simulink model "Virtual"  (Simulink 8.6)
settings: Solver=ode45  StartTime=0.0  StopTime=50.0  RelTol=1e-3
settings Model: Creator=Nasir  LastModifiedBy=Nasir
settings DebuggingCC: FcnCallInpInsideContextMsg=UseLocalSettings  StrictBusMsg=Warning
settings GRTTargetCC: GeneratePreprocessorConditionals=Use local settings
settings SimEventsCC: propDiagAttribOutput=1  propDiagFcnCallOutput=1  propDiagStatOutput=0  propPreventDuplicateEvents=0

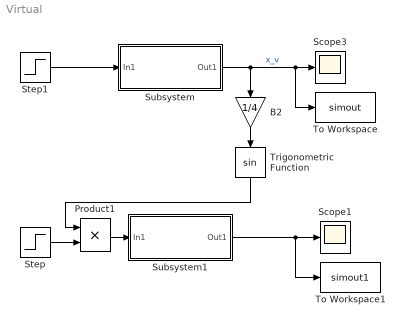
== system Virtual ==
  B2 : Gain  Gain=1/4
  Product1 : Product  RndMeth=Zero
  Scope1 : Scope
  Scope3 : Scope
  Step : Step  Before=5  After=8  SampleTime=1
  Step1 : Step  Before=4  After=8  SampleTime=0
  Subsystem : Subsystem
  Subsystem1 : Subsystem
  To Workspace : ToWorkspace  VariableName=simout  SaveFormat=Structure With Time  SampleTime=-1
  To Workspace1 : ToWorkspace  VariableName=simout1  SaveFormat=Structure With Time  SampleTime=-1
  Trigonometric Function : Trigonometry
  wires:
  Subsystem/1(Out1) -> Scope3/1, To Workspace/1, B2/1  "x_v"
  Step1/1 -> Subsystem/1(In1)
  B2/1 -> Trigonometric Function/1
  Product1/1 -> Subsystem1/1(In1)
  Subsystem1/1(Out1) -> Scope1/1, To Workspace1/1
  Step/1 -> Product1/2
  Trigonometric Function/1 -> Product1/1

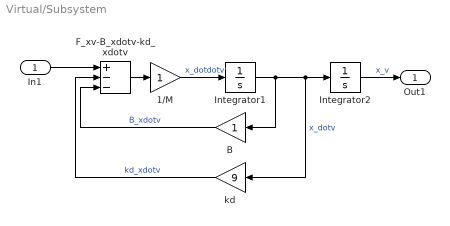
== system Virtual/Subsystem ==
  In1 : Inport
  1/M : Gain
  B : Gain
  F_xv-B_xdotv-kd_xdotv : Sum  Inputs=+--
  Integrator1 : Integrator
  Integrator2 : Integrator
  kd : Gain  Gain=9
  Out1 : Outport
  wires:
  In1/1 -> F_xv-B_xdotv-kd_xdotv/1
  Integrator1/1 -> Integrator2/1, kd/1, B/1  "x_dotv"
  kd/1 -> F_xv-B_xdotv-kd_xdotv/2  "kd_xdotv"
  F_xv-B_xdotv-kd_xdotv/1 -> 1/M/1
  B/1 -> F_xv-B_xdotv-kd_xdotv/3  "B_xdotv"
  1/M/1 -> Integrator1/1  "x_dotdotv"
  Integrator2/1 -> Out1/1  "x_v"

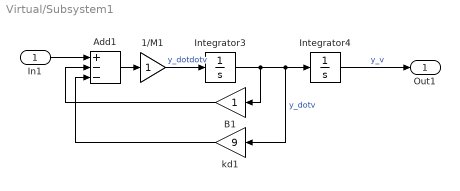
== system Virtual/Subsystem1 ==
  In1 : Inport
  1/M1 : Gain
  Add1 : Sum  Inputs=+--
  B1 : Gain
  Integrator3 : Integrator
  Integrator4 : Integrator
  kd1 : Gain  Gain=9
  Out1 : Outport
  wires:
  Integrator3/1 -> B1/1, Integrator4/1, kd1/1  "y_dotv"
  Add1/1 -> 1/M1/1
  1/M1/1 -> Integrator3/1  "y_dotdotv"
  B1/1 -> Add1/2
  kd1/1 -> Add1/3
  In1/1 -> Add1/1
  Integrator4/1 -> Out1/1  "y_v"
